simulink model "Test_simulation_model_backhoe"  (R2024a)
settings: Solver=FixedStepAuto  StartTime=0.0  StopTime=inf  FixedStep=0.0001  RelTol=1e-9
undefined symbols (not defined in the file or in its folder): X, Y, Z
libraries: sm_lib x67, nesl_utility x36, slpidlib x8
(part 4 of 4)

== matlab function Test_simulation_model_backhoe/Forward Kinematic2 ==
  data: t input; p1 output; p2 output; p3 output; p4 output
function [p1, p2, p3, p4] = FK(t)
    % FK_Simulink: Calculates the position and orientation of the end effector for a 4-DOF manipulator
    t = t;
    % Lengths of the links
    d1 = 0.3;  % {0} -> {1}
    a1 = 0.2;  % {1} -> {2}
    L1 = 0.25; % Link 1
    L2 = 1;    % Link 2
    L3 = 1.5;  % Link 3
    L4 = 0.75; % Link 4 (End Effector)

    % Extract joint angles
    % q1 = joint_angles(1); % Joint 1 (base rotation)
    % q2 = joint_angles(2); % Joint 2 (shoulder rotation)
    % q3 = joint_angles(3); % Joint 3 (elbow rotation)
    % q4 = joint_angles(4); % Joint 4 (end effector orientation)
    syms q1 q2 q3 q4

    x12 = pi/2;
    z23 = pi/2;

    % Transformation Matrices
    % Transform from base frame to end effector
    % Transformation for Joint 0 -> 1 (Rotation around the base)
    T01_T1 = [  1, 0, 0,  0;
                0, 1, 0,  0;
                0, 0, 1, d1;
                0, 0, 0,  1];

    T01_Rz = [  cos(q1), -sin(q1), 0, 0;
                sin(q1),  cos(q1), 0, 0;
                      0,        0, 1, 0;
                      0,        0, 0, 1];

    T01 = T01_T1 * T01_Rz;

    % Transformation for Joint 1 -> 2 (shoulder)
    T12_T1 = [  1, 0, 0, -a1;
                0, 1, 0,   0;
                0, 0, 1,  L1;
                0, 0, 0,   1];

    T12_Rx = [  1,        0,         0, 0;
                0, cos(x12), -sin(x12), 0;
                0, sin(x12),  cos(x12), 0;
                0,        0,         0, 1];

    T12_Rz = [  cos(q2), -sin(q2), 0, 0;
                sin(q2),  cos(q2), 0, 0;
                      0,        0, 1, 0;
                      0,        0, 0, 1];

    T12 = T12_T1 * T12_Rx * T12_Rz;

    % Transformation for Joint 2 -> 3 (elbow)
    T23_Rz1 = [  cos(z23), -sin(z23), 0, 0;
                 sin(z23),  cos(z23), 0, 0;
                        0,         0, 1, 0;
                        0,         0, 0, 1];

    T23_T1 = [  1, 0, 0, L2;
                0, 1, 0,  0;
                0, 0, 1,  0;
                0, 0, 0,  1];

    T23_Rz = [  cos(q3), -sin(q3), 0, 0;
                sin(q3),  cos(q3), 0, 0;
                      0,        0, 1, 0;
                      0,        0, 0, 1];

    T23 = T23_Rz1 * T23_T1 * T23_Rz;

    % Transformation for Joint 3 -> 4
    T34_T1 = [  1, 0, 0, L3;
                0, 1, 0,  0;
                0, 0, 1,  0;
                0, 0, 0,  1];

    T34_Rz = [  cos(q4), -sin(q4), 0, 0;
                sin(q4),  cos(q4), 0, 0;
                      0,        0, 1, 0;
                      0,        0, 0, 1];

    T34 = T34_T1 * T34_Rz;

    % Transformation for Joint 4 -> e

    T4e = [ 1, 0, 0, L4;
            0, 1, 0,  0;
            0, 0, 1,  0;
            0, 0, 0,  1];

    % Final transformation from the base to end effector
    T = T01 * T12 * T23 * T34 * T4e;
    T02 = T01 * T12;
    T03 = T02 * T23;
    T04 = T03 * T34;
    T0e = T04 * T4e;
    
    % position
    p0 = [0; 0; 0];
    p1 = T01(1:3, 4);
    p2 = T02(1:3, 4);
    p3 = T03(1:3, 4);
    p4 = T04(1:3, 4);
    pe = T0e(1:3, 4);

    % Extract position from the final transformation matrix
    x = T(1, 4); % x-position of the end effector
    y = T(2, 4); % y-position of the end effector
    z = T(3, 4); % z-position of the end effector

  
end

% Tranformation matrix
% ([  [-sin(q2 + q3 + q4)*cos(q1), -cos(q1)*cos(q2 + q3 + q4),  sin(q1), -L2*sin(q2)*cos(q1) - L3*sin(q2 + q3)*cos(q1) - L4*sin(q2 + q3 + q4)*cos(q1) - a1*cos(q1)], ...
%     [-sin(q1)*sin(q2 + q3 + q4), -sin(q1)*cos(q2 + q3 + q4), -cos(q1), -L2*sin(q1)*sin(q2) - L3*sin(q1)*sin(q2 + q3) - L4*sin(q1)*sin(q2 + q3 + q4) - a1*sin(q1)], ...
%     [         cos(q2 + q3 + q4),         -sin(q2 + q3 + q4),        0,                     L1 + L2*cos(q2) + L3*(1.0*cos(q2 + q3)) + L4*(cos(q2 + q3 + q4)) + d1], ...
%     [                         0,                          0,        0,                                                                                         1]  ])
